simulink model "High_Level_Model"  (R2024b)
settings: Solver=FixedStepAuto  StartTime=0.0  StopTime=0.1  FixedStep=.00000001  RelTol=1e-3
model workspace (MAT data in the model file):
  comp_modulation = 5
settings Model: Creator=ros  LastModifiedBy=root

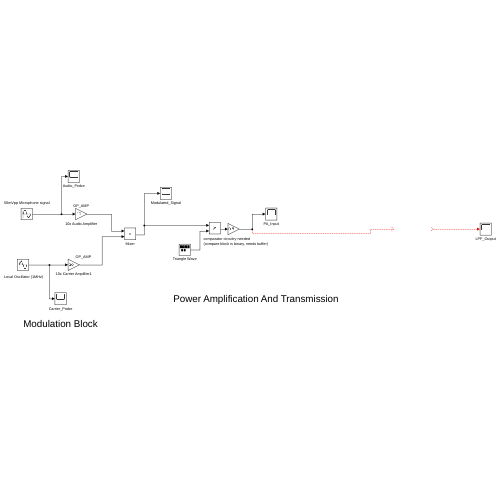
[thumbnail: Simulink's stored preview of the top-level diagram]
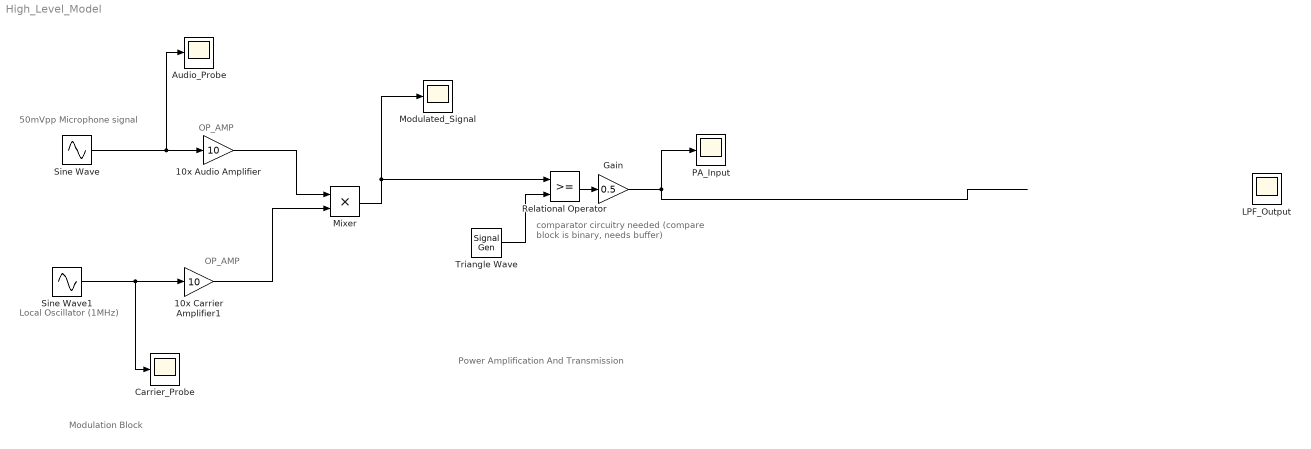
== system High_Level_Model ==
  note: comparator circuitry needed
      | (compare block is binary, needs buffer)
  note: Modulation Block
  note: OP_AMP
  note: Local Oscillator (1MHz)
  note: OP_AMP
  note: 50mVpp Microphone signal
  note: Power Amplification And Transmission
  10x Audio Amplifier : Gain  Gain=10
  10x Carrier Amplifier1 : Gain  Gain=10
  Audio_Probe : Scope
  Carrier_Probe : Scope
  Gain : Gain  Gain=0.5
  LPF_Output : Scope
  Mixer : Product
  Modulated_Signal : Scope
  PA_Input : Scope
  Relational Operator : RelationalOperator  OutDataTypeStr=boolean  RndMeth=Simplest  InputSameDT=off
  Sine Wave : Sin  Frequency=2*pi*250  SampleTime=0
  Sine Wave1 : Sin  Frequency=2*pi*1000000  SampleTime=0
  Triangle Wave : SignalGenerator  WaveForm=sawtooth  Amplitude=0.5  Frequency=1000000
  wires:
  Sine Wave/1 -> Audio_Probe/1, 10x Audio Amplifier/1
  10x Audio Amplifier/1 -> Mixer/1
  Mixer/1 -> Relational Operator/1, Modulated_Signal/1
  Sine Wave1/1 -> Carrier_Probe/1, 10x Carrier Amplifier1/1
  10x Carrier Amplifier1/1 -> Mixer/2
  Triangle Wave/1 -> Relational Operator/2
  Relational Operator/1 -> Gain/1
  Gain/1 -> PA_Input/1
  ? -> LPF_Output/1
